simulink model "trainGP_th"  (R2018b)
settings: Solver=ode45  StartTime=0.0  StopTime=simTimeGp  MaxStep=maxStep  RelTol=1e-3
values from neighbouring files (symbols this model uses):
  Cp = 0.6    [bayesian_ts.m]
  downstreamTurbPos = td*[7;0;0]    [bayesian_ts.m]    (also in wakeDeflection_ts.m)
  gpSampleInt = 10    [bayesian_ts.m]
  rhoF = 1    [bayesian_ts.m]
  rngSeed = 1    [bayesian_ts.m]
  td = 0.15    [bayesian_ts.m]    (also in wakeDeflection_ts.m)
  upstreamTurbFlow = 4    [bayesian_ts.m]    (also in wakeDeflection_ts.m)
  upstreamTurbPos = [0;0;0]    [bayesian_ts.m]    (also in wakeDeflection_ts.m)
  upstreamTurbYawSpRange = [-30 30]*pi/180    [bayesian_ts.m]
libraries: windTurbine_ul x1, gaussianProcess_ul x1, wakeDeflection_ul x1
settings Model: Creator=asiddiq2  LastModifiedBy=asiddiq2

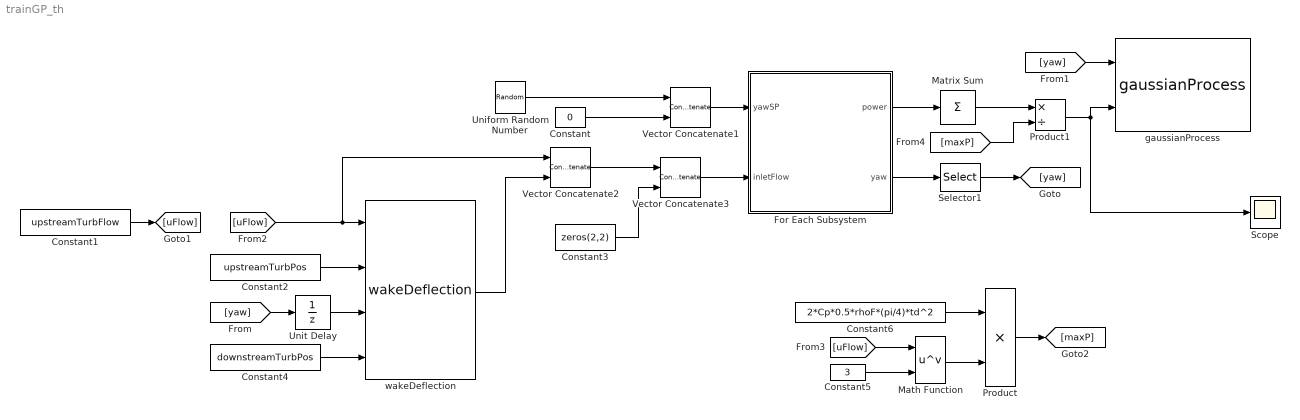
== system trainGP_th ==
  Constant : Constant  Value=0
  Constant1 : Constant  Value=upstreamTurbFlow  VectorParams1D=off
  Constant2 : Constant  Value=upstreamTurbPos  VectorParams1D=off
  Constant3 : Constant  Value=zeros(2,2)  VectorParams1D=off
  Constant4 : Constant  Value=downstreamTurbPos  VectorParams1D=off
  Constant5 : Constant  Value=3
  Constant6 : Constant  Value=2*Cp*0.5*rhoF*(pi/4)*td^2
  For Each Subsystem : Subsystem  TreatAsAtomicUnit=on
  Math Function : Math  Operator=pow  SaturateOnIntegerOverflow=on
  Matrix Sum : Sum  Inputs=+
  Product : Product
  Product1 : Product  Inputs=*/
  Scope : Scope
  Selector1 : Selector  InputPortWidth=2  IndexOptions=Index vector (dialog)  Indices=1  OutputSizes=1
  Uniform Random Number : UniformRandomNumber  Minimum=upstreamTurbYawSpRange(1)  Maximum=upstreamTurbYawSpRange(2)  Seed=rngSeed  SampleTime=1.5*gpSampleInt  VectorParams1D=off
  Unit Delay : UnitDelay  SampleTime=-1
  Vector Concatenate1 : Concatenate  Mode=Multidimensional array  ConcatenateDimension=2
  Vector Concatenate2 : Concatenate  Mode=Multidimensional array  ConcatenateDimension=2
  Vector Concatenate3 : Concatenate  Mode=Multidimensional array
  gaussianProcess : gaussianProcess_ul/gaussianProcess  dt=gpSampleInt
  wakeDeflection : wakeDeflection_ul/wakeDeflection  nTheta=nd  nD=nth  turbDia=td  ky=ky  kz=kz  CT=CT
  wires:
  For Each Subsystem/2(yaw) -> Selector1/1
  Uniform Random Number/1 -> Vector Concatenate1/1
  For Each Subsystem/1(power) -> Matrix Sum/1
  Constant4/1 -> wakeDeflection/4
  [uFlow] -> Vector Concatenate2/1, wakeDeflection/1
  Vector Concatenate1/1 -> For Each Subsystem/1(yawSP)
  Constant2/1 -> wakeDeflection/2
  Constant/1 -> Vector Concatenate1/2
  Selector1/1 -> [yaw]
  [yaw] -> gaussianProcess/1
  wakeDeflection/1 -> Vector Concatenate2/2
  Vector Concatenate2/1 -> Vector Concatenate3/1
  Vector Concatenate3/1 -> For Each Subsystem/2(inletFlow)
  Constant3/1 -> Vector Concatenate3/2
  [yaw] -> Unit Delay/1
  Constant1/1 -> [uFlow]
  [uFlow] -> Math Function/1
  Constant5/1 -> Math Function/2
  Constant6/1 -> Product/1
  Math Function/1 -> Product/2
  Product/1 -> [maxP]
  Matrix Sum/1 -> Product1/1
  Product1/1 -> gaussianProcess/2, Scope/1
  [maxP] -> Product1/2
  Unit Delay/1 -> wakeDeflection/3

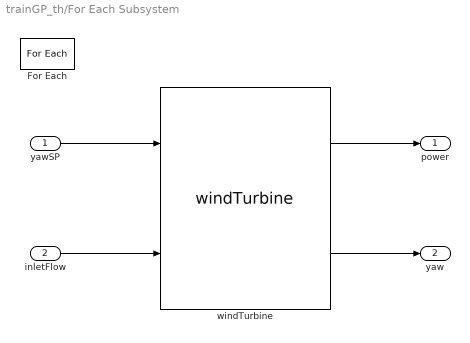
== system trainGP_th/For Each Subsystem ==
  yawSP : Inport  Partition=on  PartitionDimension=2  PartitionWidth=1  PartitionOffset=0
  inletFlow : Inport  Port=2  Partition=on  PartitionDimension=2  PartitionWidth=1  PartitionOffset=0
  For Each : ForEach  DisableCoverage=on  IndexMode=One-based
  windTurbine : windTurbine_ul/windTurbine  Cp=Cp  rhoFluid=rhoF  diam=td  Izz=Izz  iniYaw=0  gainMat=K
  power : Outport  ConcatenationDimension=2
  yaw : Outport  Port=2  ConcatenationDimension=2
  wires:
  yawSP/1 -> windTurbine/1
  inletFlow/1 -> windTurbine/2
  windTurbine/1 -> power/1
  windTurbine/2 -> yaw/1
